simulink model "Subsystem0"  (R2022b)
settings: Solver=FixedStepDiscrete  StartTime=0.0  StopTime=20.0  RelTol=1e-3  EnableMultiTasking=on
settings Model: Creator=Khaled  LastModifiedBy=Khaled
settings DataIOCC: SaveOutput=off  SaveTime=off
settings OptimizationCC: DefaultParameterBehavior=Inlined  UseDivisionForNetSlopeComputation=on  GainParamInheritBuiltInType=on  UseFloatMulNetSlope=on  InlineInvariantSignals=on  PassReuseOutputArgsAs=Individual arguments  ZeroExternalMemoryAtStartup=off  ZeroInternalMemoryAtStartup=off  NoFixptDivByZeroProtection=on  EfficientFloat2IntCast=on  LifeSpan=1  OptimizeBlockOrder=speed  DifferentSizesBufferReuse=on  EfficientTunableParamExpr=on
settings DebuggingCC: ParameterTunabilityLossMsg=error
settings HardwareCC: ProdBitPerPointer=32  ProdBitPerSizeT=32  ProdBitPerPtrDiffT=32  ProdLargestAtomicFloat=None  ProdWordSize=32  ProdLongLongMode=on  ProdHWDeviceType=Atmel->AVR (32-bit)
settings ModelReferenceCC: ModelReferenceNumInstancesAllowed=Single
settings SFSimCC: MATLABDynamicMemAlloc=off
settings RTWCC: Description=Embedded Coder  SystemTargetFile=ert.tlc  GenCodeOnly=on  TemplateMakefile=ert_default_tmf
settings CodeAppCC: ForceParamTrailComments=on  IgnoreCustomStorageClasses=off  OperatorAnnotations=on  SimulinkDataObjDesc=on  SFDataObjDesc=on  CustomSymbolStrGlobalVar=rt$N$M  CustomSymbolStrType=$N$M  CustomSymbolStrFcn=$N$M$F  CustomSymbolStrMacro=$N$M  InsertBlockDesc=on
settings ERTTargetCC: TargetLangStandard=C99 (ISO)  GenerateSampleERTMain=on  IncludeMdlTerminateFcn=off  CombineSignalStateStructs=on  SupportComplex=off  SupportNonInlinedSFcns=on  InlinedParameterPlacement=NonHierarchical  RootIOFormat=Structure reference  ERTCustomFileTemplate=example_file_process.tlc  ERTFilePackagingFormat=CompactWithDataFile

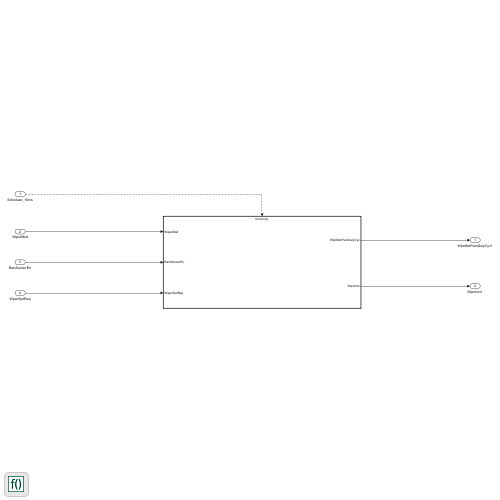
[thumbnail: Simulink's stored preview of the top-level diagram]
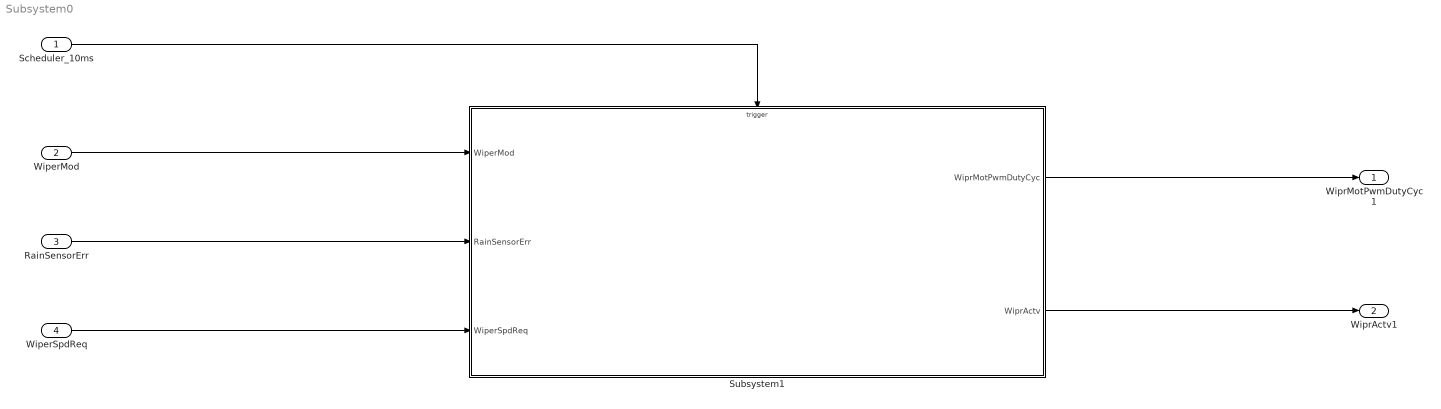
== system Subsystem0 ==
  Scheduler_10ms : Inport  PortDimensions=1  OutputFunctionCall=on
  WiperMod : Inport  Port=2  OutDataTypeStr=double  PortDimensions=1
  RainSensorErr : Inport  Port=3  OutDataTypeStr=double  PortDimensions=1
  WiperSpdReq : Inport  Port=4  OutDataTypeStr=double  PortDimensions=1
  Subsystem1 : Subsystem
  WiprMotPwmDutyCyc1 : Outport  OutDataTypeStr=double  PortDimensions=1
  WiprActv1 : Outport  Port=2  OutDataTypeStr=boolean  PortDimensions=1
  wires:
  Subsystem1/2(WiprActv) -> WiprActv1/1
  WiperMod/1 -> Subsystem1/1(WiperMod)
  Scheduler_10ms/1 -> Subsystem1/Trigger
  Subsystem1/1(WiprMotPwmDutyCyc) -> WiprMotPwmDutyCyc1/1
  RainSensorErr/1 -> Subsystem1/2(RainSensorErr)
  WiperSpdReq/1 -> Subsystem1/3(WiperSpdReq)

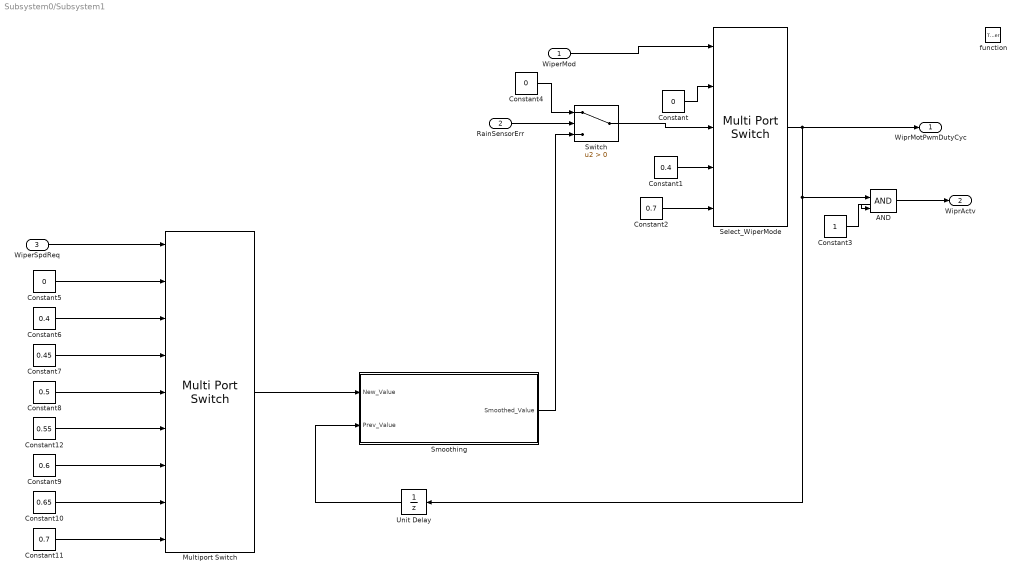
== system Subsystem0/Subsystem1 ==
  WiperMod : Inport
  RainSensorErr : Inport  Port=2
  WiperSpdReq : Inport  Port=3
  function : TriggerPort  TriggerType=function-call  VariantControl=(inherit)
  AND : Logic  IconShape=distinctive  AllPortsSameDT=off  OutDataTypeStr=boolean
  Constant : Constant  Value=0
  Constant1 : Constant  Value=0.4
  Constant10 : Constant  Value=0.65
  Constant11 : Constant  Value=0.7
  Constant12 : Constant  Value=0.55
  Constant2 : Constant  Value=0.7
  Constant3 : Constant
  Constant4 : Constant  Value=0
  Constant5 : Constant  Value=0
  Constant6 : Constant  Value=0.4
  Constant7 : Constant  Value=0.45
  Constant8 : Constant  Value=0.5
  Constant9 : Constant  Value=0.6
  Multiport Switch : MultiPortSwitch  DataPortOrder=Zero-based contiguous  Inputs=8  zeroidx=on  SaturateOnIntegerOverflow=off  InputSameDT=off
  Select_WiperMode : MultiPortSwitch  DataPortOrder=Zero-based contiguous  Inputs=4  zeroidx=on  SaturateOnIntegerOverflow=off  InputSameDT=off
  Smoothing : Subsystem
  Switch : Switch  Criteria=u2 > Threshold  OutDataTypeStr=boolean  SaturateOnIntegerOverflow=off  InputSameDT=off
  Unit Delay : UnitDelay  SampleTime=-1  HasFrameUpgradeWarning=on
  WiprMotPwmDutyCyc : Outport
  WiprActv : Outport  Port=2
  wires:
  Smoothing/1(Smoothed_Value) -> Switch/3
  Constant10/1 -> Multiport Switch/8
  Constant9/1 -> Multiport Switch/7
  Constant7/1 -> Multiport Switch/4
  Constant5/1 -> Multiport Switch/2
  Constant8/1 -> Multiport Switch/5
  Multiport Switch/1 -> Smoothing/1(New_Value)
  Constant1/1 -> Select_WiperMode/4
  Constant2/1 -> Select_WiperMode/5
  Switch/1 -> Select_WiperMode/3
  Constant/1 -> Select_WiperMode/2
  Constant12/1 -> Multiport Switch/6
  WiperSpdReq/1 -> Multiport Switch/1
  WiperMod/1 -> Select_WiperMode/1
  Constant6/1 -> Multiport Switch/3
  AND/1 -> WiprActv/1
  Unit Delay/1 -> Smoothing/2(Prev_Value)
  Select_WiperMode/1 -> Unit Delay/1, AND/1, WiprMotPwmDutyCyc/1
  Constant4/1 -> Switch/1
  RainSensorErr/1 -> Switch/2
  Constant11/1 -> Multiport Switch/9
  Constant3/1 -> AND/2

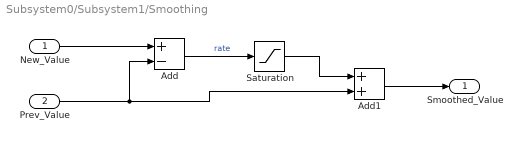
== system Subsystem0/Subsystem1/Smoothing ==
  New_Value : Inport
  Prev_Value : Inport  Port=2
  Add : Sum  Inputs=+-
  Add1 : Sum
  Saturation : Saturate  UpperLimit=0.005  LowerLimit=-0.005
  Smoothed_Value : Outport
  wires:
  Add/1 -> Saturation/1  "rate"
  New_Value/1 -> Add/1
  Prev_Value/1 -> Add1/2, Add/2
  Saturation/1 -> Add1/1
  Add1/1 -> Smoothed_Value/1
